simulink model "mass_spring_damper"  (R2022a)
settings: Solver=ode4  StartTime=0.0  StopTime=10  FixedStep=0.001  RelTol=1e-3
values from neighbouring files (symbols this model uses):
  b = 10    [mass_spring_damper_params_setup.m]
  F = 1    [mass_spring_damper_params_setup.m]
  k = 20    [mass_spring_damper_params_setup.m]
  Kd = 50    [mass_spring_damper_params_setup.m]
  Ki = 300    [mass_spring_damper_params_setup.m]
  Kp = 350    [mass_spring_damper_params_setup.m]
  M = 1    [mass_spring_damper_params_setup.m]
settings Model: Creator=stakk  LastModifiedBy=stakk

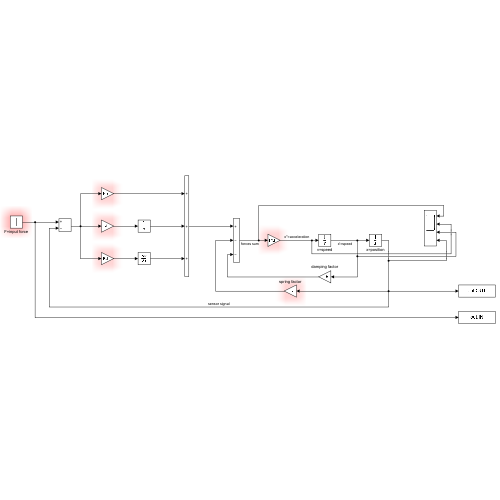
[thumbnail: Simulink's stored preview of the top-level diagram]
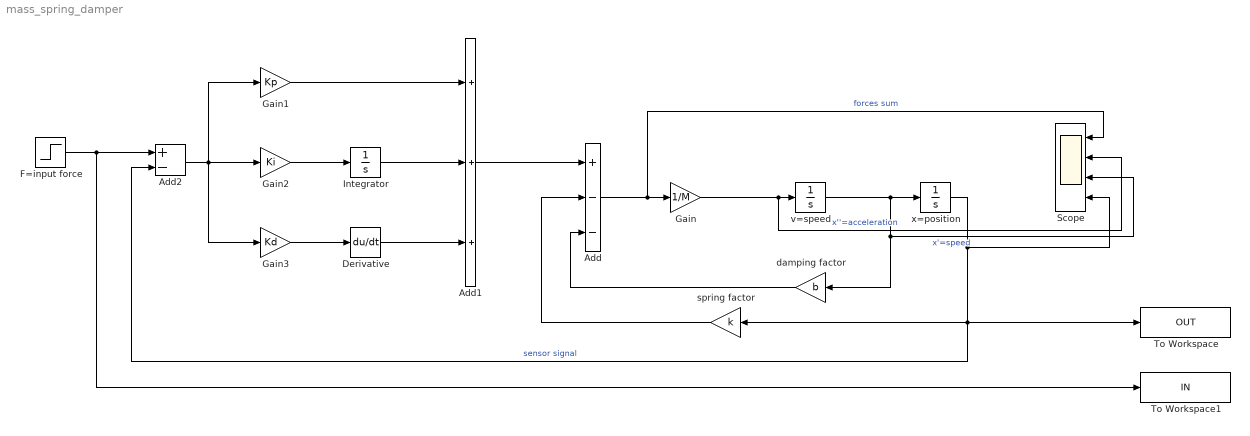
== system mass_spring_damper ==
  Add : Sum  Inputs=+--
  Add1 : Sum  Inputs=+++
  Add2 : Sum  Inputs=+-
  Derivative : Derivative
  F=input force : Step  After=F  SampleTime=0
  Gain : Gain  Gain=1/M
  Gain1 : Gain  Gain=Kp
  Gain2 : Gain  Gain=Ki
  Gain3 : Gain  Gain=Kd
  Integrator : Integrator
  Scope : Scope  NumInputPorts=4
  To Workspace : ToWorkspace  VariableName=OUT  SaveFormat=Timeseries  SampleTime=-1
  To Workspace1 : ToWorkspace  VariableName=IN  SaveFormat=Timeseries  SampleTime=-1
  damping factor : Gain  Gain=b
  spring factor : Gain  Gain=k
  v=speed : Integrator
  x=position : Integrator
  wires:
  Gain/1 -> Scope/2, v=speed/1  "x''=acceleration"
  v=speed/1 -> Scope/3, damping factor/1, x=position/1  "x'=speed"
  x=position/1 -> Scope/4, To Workspace/1, Add2/2, spring factor/1  "sensor signal"
  damping factor/1 -> Add/3
  spring factor/1 -> Add/2
  Add/1 -> Scope/1, Gain/1  "forces sum"
  Integrator/1 -> Add1/2
  Gain2/1 -> Integrator/1
  Add2/1 -> Gain1/1, Gain3/1, Gain2/1
  Derivative/1 -> Add1/3
  Gain3/1 -> Derivative/1
  Gain1/1 -> Add1/1
  Add1/1 -> Add/1
  F=input force/1 -> To Workspace1/1, Add2/1
